simulink model "traj_gen"  (R2016a)
settings: Solver=VariableStepAuto  StartTime=0.0  StopTime=0.6  RelTol=1e-3
undefined symbols (not defined in the file or in its folder): L, sigbuilder_block, T
settings Model: Creator=chao  LastModifiedBy=chao

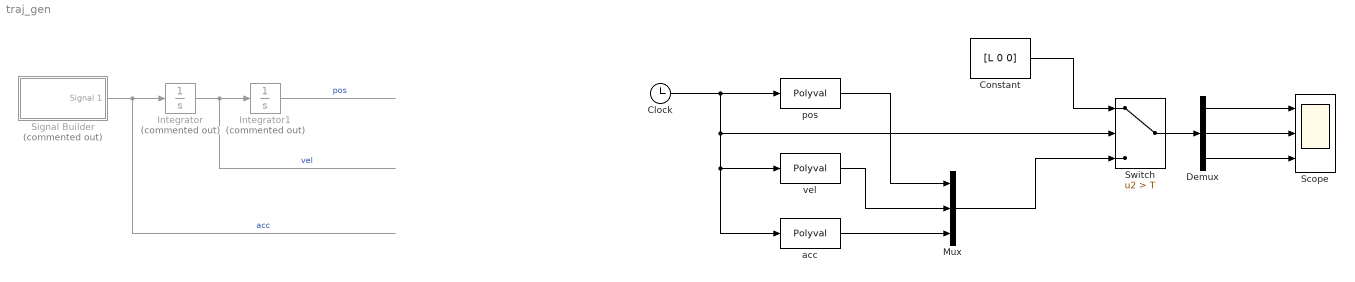
== system traj_gen ==
  Clock : Clock
  Constant : Constant  Value=[L 0 0]
  Demux : Demux  Outputs=3
  Integrator : Integrator  Commented=on
  Integrator1 : Integrator  Commented=on
  Mux : Mux  Inputs=3
  Scope : Scope  NumInputPorts=3
  Signal Builder : Subsystem  Tag=STV Subsys  Commented=on  LoadFcn=sigbuilder_block('load');  StartFcn=sigbuilder_block('start');  StopFcn=sigbuilder_block('stop');  ClipboardFcn=sigbuilder_block('clipboard');  mask(Sigbuilder block){}
      mask help: Simulink:masks:SigbuilderBlock_MD
      mask init:
      | if ~strcmp(get_param(bdroot(gcbh),'SimulationStatus'),'stopped') tuvar = sigbuilder_block('maskInit'); end
      settings: CopyFcn=sigbuilder_block('copy');  DeleteFcn=sigbuilder_block('delete');  ModelCloseFcn=sigbuilder_block('modelClose');  PreSaveFcn=sigbuilder_block('preSave');  PauseFcn=sigbuilder_block('pause');  ContinueFcn=sigbuilder_block('continue');  NameChangeFcn=sigbuilder_block('namechange');  OpenFcn=sigbuilder_block('open',[436.2 135.6 550.8 400.2 ]);  CloseFcn=sigbuilder_block('close');
      mask Display: plot(0, 0, 100, 100,[2, 2, 32, 32, 2], [68, 8, 8, 68, 68],[32, 2], [38, 38], [32, 19, 2],[53, 60, 44], [32, 17, 17, 2],[16, 16, 31, 31]);txt = getActiveGroup(gcbh);text(2, 100, txt,'verticalAlignment', 'top');
  Switch : Switch  Criteria=u2 > Threshold  Threshold=T
  acc : Polyval  Coefs=[120*L/(T^5), -180*L/(T^4), 60*L/(T^3), 0]
  pos : Polyval  Coefs=[6*L/(T^5), -15*L/(T^4), 10*L/(T^3), 0, 0, 0]
  vel : Polyval  Coefs=[30*L/(T^5), -60*L/(T^4), 30*L/(T^3), 0, 0]
  wires:
  Signal Builder/1(Signal 1) -> Integrator/1  "acc"
  Integrator/1 -> Integrator1/1  "vel"
  Integrator1/1 -> ?  "pos"
  Clock/1 -> acc/1, vel/1, Switch/2, pos/1
  pos/1 -> Mux/1
  vel/1 -> Mux/2
  acc/1 -> Mux/3
  Mux/1 -> Switch/3
  Constant/1 -> Switch/1
  Switch/1 -> Demux/1
  Demux/2 -> Scope/2
  Demux/1 -> Scope/1
  Demux/3 -> Scope/3

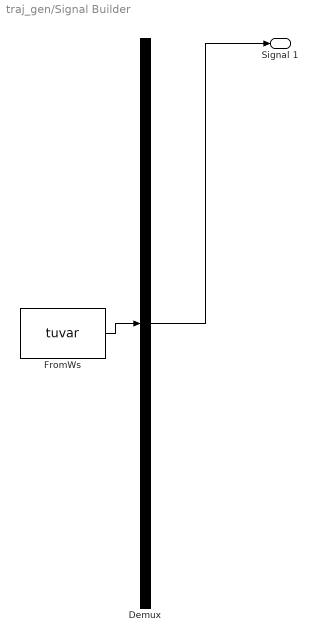
== system traj_gen/Signal Builder ==
  Demux : Demux  Tag=STV Demux  Outputs=1
  FromWs : FromWorkspace  Tag=STV FromWs  VariableName=tuvar  SampleTime=0
      SigBuilderData=|
      | common.afterFinalStr = 'Extrapolate'
      | common.sampleTime = 0
      | dataSet.timeRange = [0 1]
      | dataSet.name = 'Group 1'
      | sbobj.Groups.Name = 'Group 1'
      | sbobj.Groups.Signals.Name = 'Signal 1'
      | sbobj.Groups.Signals.XData = [0 0.1 0.1 0.3 0.3 0.4 0.4 1]
      | sbobj.Groups.Signals.YData = [3.3 3.3 0 0 -3.3 -3.3 0 0]
      | sbobj.Groups.TimeRange = [0 1]
  Signal 1 : Outport  Tag=STV Outport
  wires:
  Demux/1 -> Signal 1/1
  FromWs/1 -> Demux/1
